simulink model "ComplianceControl"  (R2023a)
settings: Solver=VariableStepAuto  StartTime=0.0  StopTime=app.StopTime  RelTol=1e-3
undefined symbols (not defined in the file or in its folder): app, forwardKinematics, Generate_G, GenerateAnlyticalJacobian, TrimUnusedDofs_rows
settings Model: Creator=Ericw  LastModifiedBy=wgrie

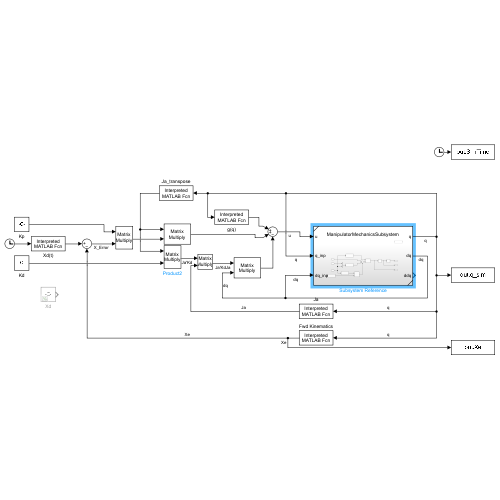
[thumbnail: Simulink's stored preview of the top-level diagram]
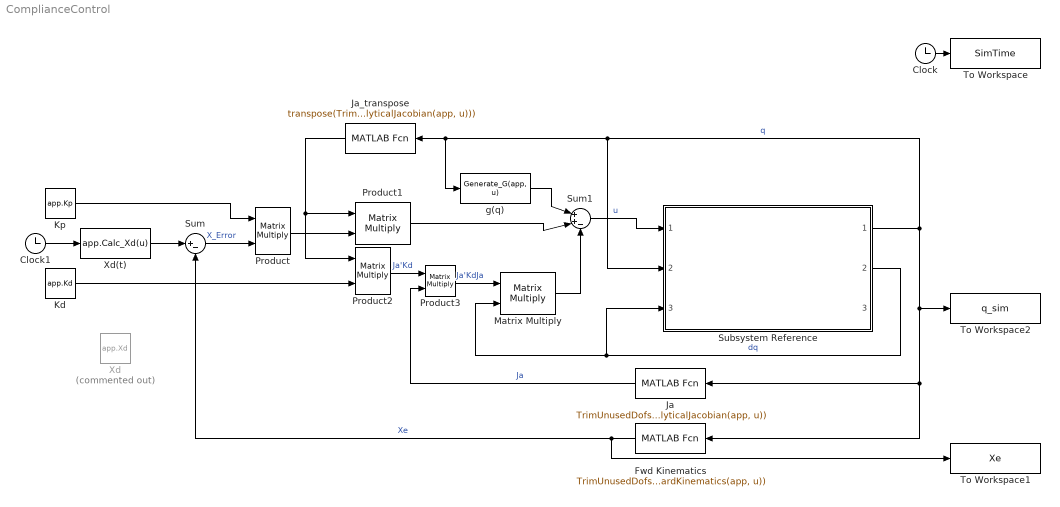
== system ComplianceControl ==
  Clock : Clock
  Clock1 : Clock
  Fwd Kinematics : MATLABFcn  MATLABFcn=TrimUnusedDofs_rows(app,forwardKinematics(app, u))  OutputDimensions=[app.numActiveDofs,1]  Output1D=off
  Ja : MATLABFcn  MATLABFcn=TrimUnusedDofs_rows(app,GenerateAnlyticalJacobian(app, u))  OutputDimensions=[app.numActiveDofs,app.NumJoints]  Output1D=off
  Ja_transpose : MATLABFcn  MATLABFcn=transpose(TrimUnusedDofs_rows(app, GenerateAnlyticalJacobian(app, u)))  OutputDimensions=[app.NumJoints,app.numActiveDofs]  Output1D=off
  Kd : Constant  Value=app.Kd
  Kp : Constant  Value=app.Kp
  Matrix Multiply : Product  Multiplication=Matrix(*)
  Product{,1..3} (4 alike) : Product  Multiplication=Matrix(*)
  Subsystem Reference : Subsystem  ReferencedSubsystem=ManipulatorMechanicsSubsystem
  Sum : Sum  Inputs=|+-
  Sum1 : Sum  Inputs=|++-
  To Workspace : ToWorkspace  VariableName=SimTime  SaveFormat=Timeseries  SampleTime=-1
  To Workspace1 : ToWorkspace  VariableName=Xe  SaveFormat=Timeseries  SampleTime=-1
  To Workspace2 : ToWorkspace  VariableName=q_sim  SaveFormat=Timeseries  SampleTime=-1
  Xd : Constant  Commented=on  Value=app.Xd  VectorParams1D=off
  Xd(t) : MATLABFcn  MATLABFcn=app.Calc_Xd(u)  OutputDimensions=[app.numActiveDofs,1]  Output1D=off
  g(q) : MATLABFcn  MATLABFcn=Generate_G(app, u)  OutputDimensions=[app.NumJoints,1]  Output1D=off
  wires:
  Sum/1 -> Product/2  "X_Error"
  Kp/1 -> Product/1
  Subsystem Reference/1 -> Ja_transpose/1, g(q)/1, Subsystem Reference/2, To Workspace2/1, Fwd Kinematics/1, Ja/1  "q"
  Product/1 -> Product1/2
  Ja_transpose/1 -> Product2/1, Product1/1
  Subsystem Reference/2 -> Matrix Multiply/2, Subsystem Reference/3  "dq"
  Product1/1 -> Sum1/2
  g(q)/1 -> Sum1/1
  Sum1/1 -> Subsystem Reference/1  "u"
  Kd/1 -> Product2/2
  Product2/1 -> Product3/1  "Ja'Kd"
  Ja/1 -> Product3/2  "Ja"
  Fwd Kinematics/1 -> To Workspace1/1, Sum/2  "Xe"
  Clock/1 -> To Workspace/1
  Product3/1 -> Matrix Multiply/1  "Ja'KdJa"
  Matrix Multiply/1 -> Sum1/3
  Clock1/1 -> Xd(t)/1
  Xd(t)/1 -> Sum/1
